simulink model "Control_ETHERLAB_2018b"  (R2018b)
settings: Solver=FixedStepDiscrete  StartTime=0.0  StopTime=inf  FixedStep=0.001  RelTol=1e-3
PreLoadFcn:
  | addpath(genpath('/opt/etherlab'))
InitFcn:
  | addpath(genpath('/opt/etherlab'))
undefined symbols (not defined in the file): motor_ec1
libraries: dspindex x10, dspfdesign x3
settings Model: SimulationMode=external  ExtModeTrigDuration=100  ExtModeArchiveFileName=measurement_data  ExtModeArchiveDirName=/home/cybathalon/Documents/Motor_test/Data/  Creator=schappler  LastModifiedBy=Rossgoderer
settings DataIOCC: SaveFormat=StructureWithTime  SaveOutput=off  SignalLogging=off  SaveTime=off
settings OptimizationCC: BlockReduction=off  ConditionallyExecuteInputs=off  OptimizeBlockIOStorage=off  BufferReuse=off  GlobalBufferReuse=off  ExpressionFolding=off  LocalBlockOutputs=off  OptimizeDataStoreBuffers=off  BusAssignmentInplaceUpdate=off
settings DebuggingCC: InheritedTsInSrcMsg=none
settings HardwareCC: ProdBitPerPointer=32  ProdBitPerSizeT=32  ProdBitPerPtrDiffT=32  ProdLargestAtomicInteger=Long  ProdWordSize=32  ProdHWDeviceType=ARM Compatible->ARM 10
settings SFSimCC: SimUseLocalCustomCode=off
settings RTWCC: Description=EtherLab PREEMT_RT Real-Time Target  SystemTargetFile=etherlab.tlc  PackageName=test  TemplateMakefile=etherlab_hrt.tmf  RTWUseLocalCustomCode=off
settings CodeAppCC: StateflowObjectComments=on
settings STFCustomTargetCC: TargetLangStandard=C99 (ISO)  GRTInterface=on  SystemTargetFile=etherlab.tlc
settings GRTTargetCC: ParMdlRefBuildCompliant=off  CompOptLevelCompliant=off  ConcurrentExecutionCompliant=off  CombineOutputUpdateFcns=off  MatFileLogging=off  CPPClassGenCompliant=off  GRTInterface=on  UseToolchainInfoCompliant=off  ExtMode=on  ExtModeStaticAlloc=on  ExtModeStaticAllocSize=10000000  ExtModeMexArgs='localhost' 0 17725  RTWCAPISignals=on  RTWCAPIParams=on
settings SimscapeCC: SimscapeNormalizeSystem=off

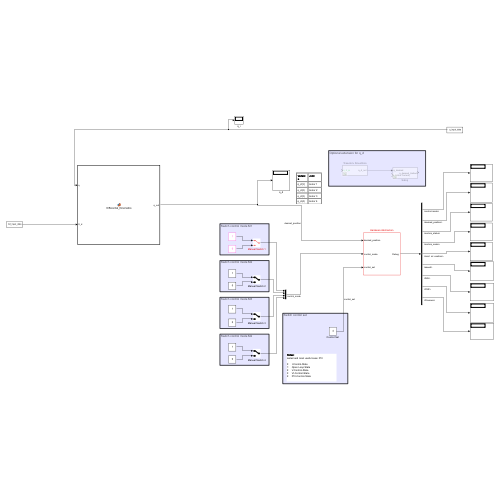
[thumbnail: Simulink's stored preview of the top-level diagram]
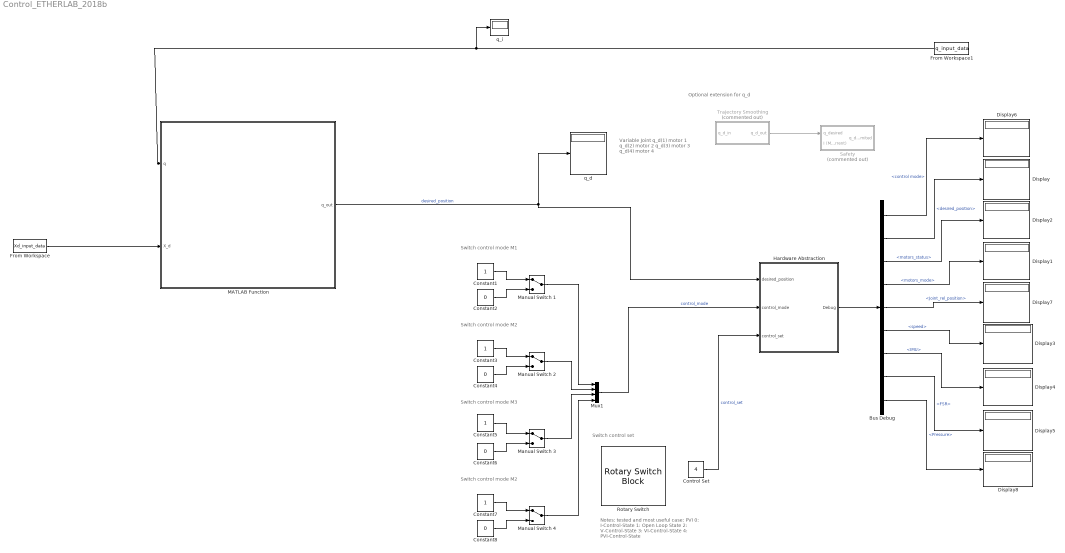
== system Control_ETHERLAB_2018b ==
  note: Optional extension for q_d
  note: Switch control mode M1
  note: Variable
      | Joint
      |
      | q_d(1)
      |
      | motor 1
      |
      | q_d(2)
      | motor 2
      |
      | q_d(3)
      | motor 3
      |
      | q_d(4)
      | motor 4
  note: Switch control mode M2
  note: Switch control mode M3
  note: Switch control mode M2
  note: Switch control set
  note: Notes:
      | tested and most useful case: PVI
      |
      | 0: I-Control-State
      | 1: Open Loop State
      | 2: V-Control-State
      | 3: VI-Control-State
      | 4: PVI-Control-State
  Bus Debug : BusSelector  OutputSignals=control mode,desired_position,motors_status,motors_mode,Joint_rel_position,speed,IMU,FSR,Pressure
  Constant{1,3,5,7} (4 alike) : Constant  VectorParams1D=off
  Constant{2,4,6,8} (4 alike) : Constant  Value=0  VectorParams1D=off
  Control Set : Constant  Value=4  VectorParams1D=off
  Display{,1..8} (9 alike) : Display
  From Workspace : FromWorkspace  VariableName=Xd_input_data  SampleTime=0.01  Interpolate=off  OutputAfterFinalValue=Setting to zero
  From Workspace1 : FromWorkspace  VariableName=q_input_data  SampleTime=0.01  Interpolate=off  OutputAfterFinalValue=Setting to zero
  Hardware Abstraction : Subsystem
  MATLAB Function : MATLAB Function  TreatAsAtomicUnit=on
  Manual Switch {1..4} (4 alike) : ManualSwitch
  Mux1 : Mux
  Rotary Switch : RotarySwitchBlock  WebBlockId=10885
      settings: Values={{'I', 'OL', 'V', 'VI', 'PVI'}, [0 1 2 3 4]}
  Safety : Subsystem  Commented=on
  Trajectory Smoothing : Subsystem  Commented=on
  q_d : Display
      settings: Description=|
      | Wrist
      | Gripper
  "q_i " : Display
      settings: Description=|
      | Wrist
      | Gripper
  wires:
  Trajectory Smoothing/1(q_d_out) -> Safety/1(q_desired)
  Hardware Abstraction/1("Debug ") -> Bus Debug/1
  Bus Debug/2 -> Display/1  "<desired_position>"
  Bus Debug/4 -> Display1/1  "<motors_mode>"
  Bus Debug/6 -> Display3/1  "<speed>"
  Bus Debug/1 -> Display6/1  "<control mode>"
  Bus Debug/5 -> Display7/1  "<Joint_rel_position>"
  Constant1/1 -> Manual Switch 1/1
  Constant2/1 -> Manual Switch 1/2
  Manual Switch 1/1 -> Mux1/1
  Mux1/1 -> Hardware Abstraction/2(control_mode)  "control_mode"
  Manual Switch 2/1 -> Mux1/2
  Constant4/1 -> Manual Switch 2/2
  Constant3/1 -> Manual Switch 2/1
  Constant5/1 -> Manual Switch 3/1
  Constant6/1 -> Manual Switch 3/2
  Manual Switch 3/1 -> Mux1/3
  Constant7/1 -> Manual Switch 4/1
  Constant8/1 -> Manual Switch 4/2
  Manual Switch 4/1 -> Mux1/4
  Control Set/1 -> Hardware Abstraction/3(control_set)  "control_set"
  Bus Debug/3 -> Display2/1  "<motors_status>"
  Bus Debug/7 -> Display4/1  "<IMU>"
  Bus Debug/8 -> Display5/1  "<FSR>"
  Bus Debug/9 -> Display8/1  "<Pressure>"
  MATLAB Function/1(q_out) -> Hardware Abstraction/1(desired_position), q_d/1  "desired_position"
  From Workspace/1 -> MATLAB Function/2(X_d)
  From Workspace1/1 -> "q_i "/1, MATLAB Function/1(q)

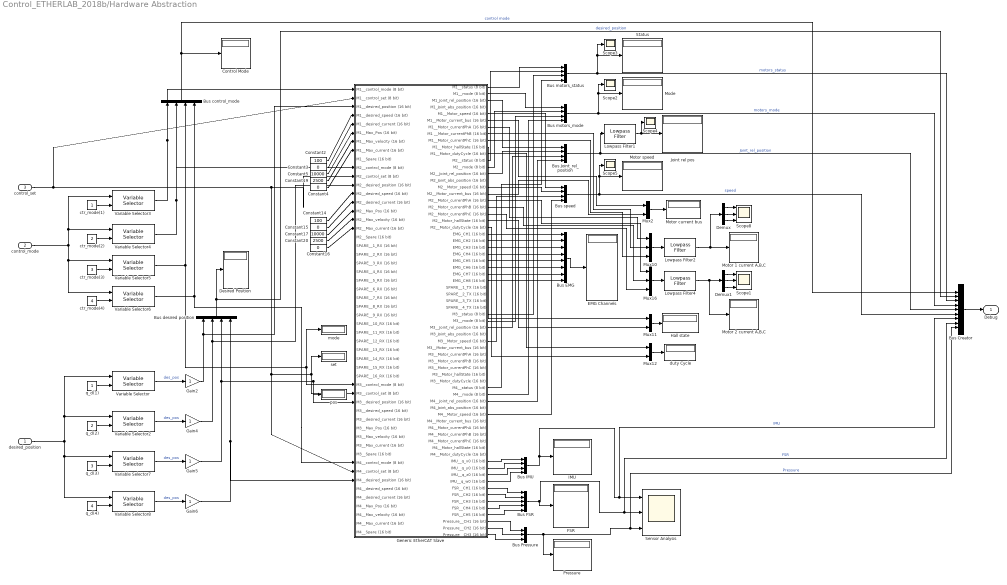
== system Control_ETHERLAB_2018b/Hardware Abstraction ==
  desired_position : Inport
  control_mode : Inport  Port=2
  control_set : Inport  Port=3
  Bus Creator : BusCreator  Inputs=9
  Bus EMG : BusCreator  Inputs=8
  Bus FSR : BusCreator  Inputs=5
  Bus IMU : BusCreator  Inputs=4
  Bus Joint_rel_position : BusCreator  Inputs=4
  Bus Pressure : BusCreator  Inputs=3
  Bus control_mode : BusCreator  Inputs=4
  Bus desired position : BusCreator  Inputs=4
  Bus motors_mode : BusCreator  Inputs=4
  Bus motors_status : BusCreator  Inputs=4
  Bus speed : BusCreator  Inputs=4
  Constant14 : Constant  Value=100
  Constant{3..4,15..16} (4 alike) : Constant  Value=0
  Constant17 : Constant  Value=10000
  Constant19 : Constant  Value=2500
  Constant2 : Constant  Value=100
  Constant20 : Constant  Value=2500
  Constant5 : Constant  Value=10000
  Control Mode : Display
  Demux : Demux  Outputs=3
  Demux1 : Demux  Outputs=3
  Desired Position : Display
  EMG Channels : Display
  FSR : Display
  Gain{2,4..6} (4 alike) : Gain
  Generic EtherCAT Slave : Subsystem
  Hall state : Display
  IMU : Display
  Joint rel pos : Display
  Lowpass Filter1 : dspfdesign/Lowpass Filter  FilterType=FIR  DesignForMinimumOrder=on  FilterOrder=50  PassbandFrequency=1  StopbandFrequency=10  PassbandRipple=0.1  StopbandAttenuation=10  InheritSampleRate=off  SampleRate=1000  SimulateUsing=Interpreted execution  roundingMode=Floor  coeffsDataTypeStr=fixdt(1,16)
  Lowpass Filter2 : dspfdesign/Lowpass Filter  FilterType=FIR  DesignForMinimumOrder=on  FilterOrder=50  PassbandFrequency=1  StopbandFrequency=10  PassbandRipple=0.1  StopbandAttenuation=80  InheritSampleRate=off  SampleRate=1000  SimulateUsing=Interpreted execution  roundingMode=Floor  coeffsDataTypeStr=fixdt(1,16)
  Lowpass Filter4 : dspfdesign/Lowpass Filter  FilterType=FIR  DesignForMinimumOrder=on  FilterOrder=50  PassbandFrequency=1  StopbandFrequency=10  PassbandRipple=0.1  StopbandAttenuation=80  InheritSampleRate=off  SampleRate=1000  SimulateUsing=Interpreted execution  roundingMode=Floor  coeffsDataTypeStr=fixdt(1,16)
  Mode : Display
  Motor 1 current A,B,C : Display
  Motor 2 current A,B,C : Display
  Motor current bus : Display
  Motor speed : Display
  Mux10 : Mux  Inputs=3
  Mux11 : Mux  Inputs=2
  Mux12 : Mux  Inputs=2
  Mux16 : Mux  Inputs=3
  Mux2 : Mux  Inputs=2
  Pressure : Display
  Scope1 : Scope  NumInputPorts=3
  Scope{2..5} (4 alike) : Scope
  Scope8 : Scope  NumInputPorts=3
  Sensor Analysis : Scope  NumInputPorts=3
  Status : Display
  Variable Selector{,2..8} (8 alike) : dspindex/Variable Selector  NumInputs=1  rowsOrCols=Rows  IdxMode=Variable  Elements=[1 3]  ZerOneIdxMode=One-based  errmode=Clip Index  FillMode=on  FillValues=0
  ctr_mode(1) : Constant  SampleTime=-1
  ctr_mode(2) : Constant  Value=2  SampleTime=-1
  ctr_mode(3) : Constant  Value=3  SampleTime=-1
  ctr_mode(4) : Constant  Value=4  SampleTime=-1
  duty Cycle : Display
  mode : Display
  pos : Display
  q_d(1) : Constant  SampleTime=-1
  q_d(2) : Constant  Value=2  SampleTime=-1
  q_d(3) : Constant  Value=3  SampleTime=-1
  q_d(4) : Constant  Value=4  SampleTime=-1
  "set " : Display
  "Debug " : Outport  VectorParamsAs1DForOutWhenUnconnected=off
  wires:
  Variable Selector/1 -> Gain2/1  "des_pos"
  q_d(1)/1 -> Variable Selector/2
  Bus motors_status/1 -> Scope3/1, Status/1, Bus Creator/3  "motors_status"
  Bus Creator/1 -> "Debug "/1
  q_d(2)/1 -> Variable Selector2/2
  Variable Selector2/1 -> Gain4/1  "des_pos"
  ctr_mode(1)/1 -> Variable Selector3/2
  ctr_mode(2)/1 -> Variable Selector4/2
  Bus EMG/1 -> EMG Channels/1
  Generic EtherCAT Slave/23(EMG_CH1 (16 bit)) -> Bus EMG/1
  Generic EtherCAT Slave/24(EMG_CH2 (16 bit)) -> Bus EMG/2
  Generic EtherCAT Slave/25(EMG_CH3 (16 bit)) -> Bus EMG/3
  Generic EtherCAT Slave/26(EMG_CH4 (16 bit)) -> Bus EMG/4
  Generic EtherCAT Slave/27(EMG_CH5 (16 bit)) -> Bus EMG/5
  Generic EtherCAT Slave/28(EMG_CH6 (16 bit)) -> Bus EMG/6
  Generic EtherCAT Slave/29(EMG_CH7 (16 bit)) -> Bus EMG/7
  Generic EtherCAT Slave/30(EMG_CH8 (16 bit)) -> Bus EMG/8
  Generic EtherCAT Slave/2(M1__mode (8 bit)) -> Bus motors_mode/1
  Generic EtherCAT Slave/1(M1__status (8 bit)) -> Bus motors_status/1
  Generic EtherCAT Slave/12(M2__status (8 bit)) -> Bus motors_status/2
  Generic EtherCAT Slave/13(M2__mode (8 bit)) -> Bus motors_mode/2
  Generic EtherCAT Slave/14(M2__Joint_rel_position (16 bit)) -> Bus Joint_rel_position/2
  Mux2/1 -> Motor current bus/1
  Mux10/1 -> Lowpass Filter2/1
  Generic EtherCAT Slave/6(M1__Motor_current_bus (16 bit)) -> Mux2/1
  Generic EtherCAT Slave/17(M2__Motor_current_bus (16 bit)) -> Mux2/2
  Generic EtherCAT Slave/7(M1__Motor_currentPhA (16 bit)) -> Mux10/1
  Generic EtherCAT Slave/8(M1 __Motor_currentPhB (16 bit)) -> Mux10/2
  Generic EtherCAT Slave/9(M1__Motor_currentPhC (16 bit)) -> Mux10/3
  Generic EtherCAT Slave/18(M2__Motor_currentPhA (16 bit)) -> Mux16/1
  Generic EtherCAT Slave/19(M2__Motor_currentPhB (16 bit)) -> Mux16/2
  Generic EtherCAT Slave/20(M2__Motor_currentPhC (16 bit)) -> Mux16/3
  Mux11/1 -> Hall state/1
  Generic EtherCAT Slave/10(M1__Motor_hallState (16 bit)) -> Mux11/1
  Generic EtherCAT Slave/21(M2__Motor_hallState (16 bit)) -> Mux11/2
  Mux12/1 -> duty Cycle/1
  Generic EtherCAT Slave/11(M1__Motor_dutyCycle (16 bit)) -> Mux12/1
  Generic EtherCAT Slave/22(M2__Motor_dutyCycle (16 bit)) -> Mux12/2
  Bus IMU/1 -> Sensor Analysis/1, Bus Creator/7, IMU/1  "IMU"
  Generic EtherCAT Slave/57(IMU__q_x0 (16 bit)) -> Bus IMU/1
  Generic EtherCAT Slave/58(IMU__q_y0 (16 bit)) -> Bus IMU/2
  Generic EtherCAT Slave/59(IMU__q_z0 (16 bit)) -> Bus IMU/3
  Generic EtherCAT Slave/60(IMU__q_w0 (16 bit)) -> Bus IMU/4
  Generic EtherCAT Slave/64(FSR__CH4 (16 bit)) -> Bus FSR/4
  Generic EtherCAT Slave/61(FSR__CH1 (16 bit)) -> Bus FSR/1
  Generic EtherCAT Slave/63(FSR__CH3 (16 bit)) -> Bus FSR/3
  Generic EtherCAT Slave/62(FSR__CH2 (16 bit)) -> Bus FSR/2
  Generic EtherCAT Slave/65(FSR__CH5 (16 bit)) -> Bus FSR/5
  Bus Pressure/1 -> Bus Creator/9, Sensor Analysis/3, Pressure/1  "Pressure"
  Generic EtherCAT Slave/66(Pressure__CH1 (16 bit)) -> Bus Pressure/1
  Generic EtherCAT Slave/67(Pressure__CH2 (16 bit)) -> Bus Pressure/2
  Generic EtherCAT Slave/68(Pressure__CH3 (16 bit)) -> Bus Pressure/3
  Variable Selector3/1 -> Generic EtherCAT Slave/1(M1__control_mode (8 bit)), Bus control_mode/1
  Constant14/1 -> Generic EtherCAT Slave/13(M2__desired_speed (16 bit))
  Constant15/1 -> Generic EtherCAT Slave/14(M2__desired_current (16 bit))
  Gain4/1 -> Generic EtherCAT Slave/12(M2__desired_position (16 bit)), Bus desired position/2
  Variable Selector4/1 -> Generic EtherCAT Slave/10(M2__control_mode (8 bit)), Bus control_mode/2
  control_set/1 -> Generic EtherCAT Slave/45(M4__control_set (8 bit)), "set "/1, Generic EtherCAT Slave/36(M3__control_set (8 bit)), Generic EtherCAT Slave/11(M2__control_set (8 bit)), Generic EtherCAT Slave/2(M1__control_set (8 bit))
  Constant2/1 -> Generic EtherCAT Slave/4(M1__desired_speed (16 bit))
  Constant19/1 -> Generic EtherCAT Slave/7(M1__Max_velocity (16 bit))
  Gain2/1 -> Generic EtherCAT Slave/3(M1__desired_position (16 bit)), Bus desired position/1
  Constant5/1 -> Generic EtherCAT Slave/6(M1__Max_Pos (16 bit))
  Constant3/1 -> Generic EtherCAT Slave/5(M1__desired_current (16 bit))
  Constant4/1 -> Generic EtherCAT Slave/8(M1__Max_current (16 bit))
  Lowpass Filter2/1 -> Demux/1, Motor 1 current A,B,C/1
  Mux16/1 -> Lowpass Filter4/1
  Lowpass Filter4/1 -> Demux1/1, Motor 2 current A,B,C/1
  ctr_mode(3)/1 -> Variable Selector5/2
  ctr_mode(4)/1 -> Variable Selector6/2
  control_mode/1 -> Variable Selector3/1, Variable Selector4/1, Variable Selector6/1, Variable Selector5/1
  Variable Selector5/1 -> Bus control_mode/3, mode/1, Generic EtherCAT Slave/35(M3__control_mode (8 bit))
  Variable Selector6/1 -> Bus control_mode/4, Generic EtherCAT Slave/44(M4__control_mode (8 bit))
  Bus control_mode/1 -> Bus Creator/1, Control Mode/1  "control mode"
  q_d(3)/1 -> Variable Selector7/2
  desired_position/1 -> Variable Selector2/1, Variable Selector/1, Variable Selector8/1, Variable Selector7/1
  q_d(4)/1 -> Variable Selector8/2
  Variable Selector7/1 -> Gain5/1  "des_pos"
  Variable Selector8/1 -> Gain6/1  "des_pos"
  Gain5/1 -> pos/1, Generic EtherCAT Slave/37(M3__desired_position (16 bit)), Bus desired position/3
  Gain6/1 -> Generic EtherCAT Slave/46(M4__desired_position (16 bit)), Bus desired position/4
  Bus desired position/1 -> Desired Position/1, Bus Creator/2  "desired_position"
  Demux/1 -> Scope8/1
  Demux/2 -> Scope8/2
  Demux/3 -> Scope8/3
  Demux1/3 -> Scope1/3
  Demux1/2 -> Scope1/2
  Demux1/1 -> Scope1/1
  Generic EtherCAT Slave/35(M3__status (8 bit)) -> Bus motors_status/3
  Generic EtherCAT Slave/46(M4__status (8 bit)) -> Bus motors_status/4
  Generic EtherCAT Slave/36(M3__mode (8 bit)) -> Bus motors_mode/3
  Generic EtherCAT Slave/47(M4__mode (8 bit)) -> Bus motors_mode/4
  Bus motors_mode/1 -> Bus Creator/4, Scope2/1, Mode/1  "motors_mode"
  Generic EtherCAT Slave/3(M1_Joint_rel_position (16 bit)) -> Bus Joint_rel_position/1
  Generic EtherCAT Slave/37(M3__Joint_rel_position (16 bit)) -> Bus Joint_rel_position/3
  Generic EtherCAT Slave/48(M4__Joint_rel_position (16 bit)) -> Bus Joint_rel_position/4
  Bus Joint_rel_position/1 -> Lowpass Filter1/1, Bus Creator/5  "Joint_rel_position"
  Bus speed/1 -> Bus Creator/6, Scope5/1, Motor speed/1  "speed"
  Generic EtherCAT Slave/5(M1__Motor_speed (16 bit)) -> Bus speed/1
  Generic EtherCAT Slave/16(M2__Motor_speed (16 bit)) -> Bus speed/2
  Generic EtherCAT Slave/39(M3__Motor_speed (16 bit)) -> Bus speed/3
  Generic EtherCAT Slave/50(M4__Motor_speed (16 bit)) -> Bus speed/4
  Bus FSR/1 -> Sensor Analysis/2, Bus Creator/8, FSR/1  "FSR"
  Constant17/1 -> Generic EtherCAT Slave/15(M2__Max_Pos (16 bit))
  Constant20/1 -> Generic EtherCAT Slave/16(M2__Max_velocity (16 bit))
  Constant16/1 -> Generic EtherCAT Slave/17(M2__Max_current (16 bit))
  Lowpass Filter1/1 -> Scope4/1, Joint rel pos/1

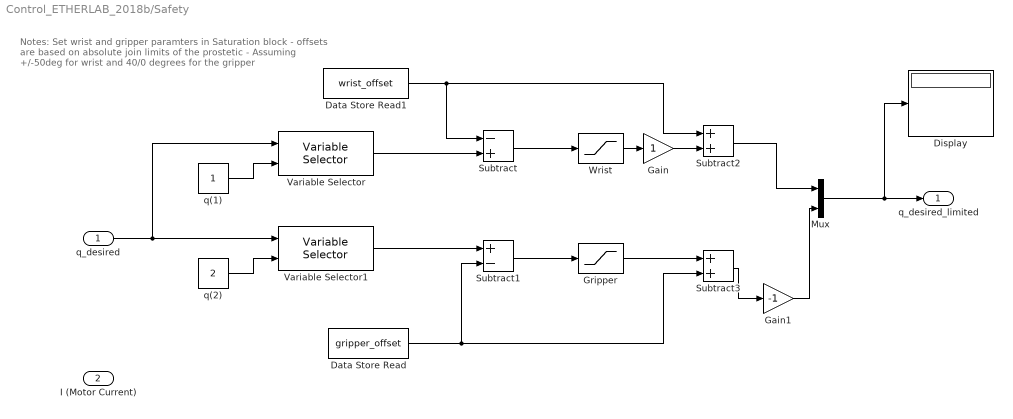
== system Control_ETHERLAB_2018b/Safety ==
  note: Notes:
      | Set wrist and gripper paramters in Saturation block
      | - offsets are based on absolute join limits of the prostetic
      | - Assuming +/-50deg for wrist and 40/0 degrees for the gripper
  q_desired : Inport
  I (Motor Current) : Inport  Port=2
  Data Store Read : DataStoreRead  DataStoreName=gripper_offset  DataStoreElements=gripper_offset
  Data Store Read1 : DataStoreRead  DataStoreName=wrist_offset  DataStoreElements=wrist_offset
  Display : Display
  Gain : Gain
  Gain1 : Gain  Gain=-1
  Gripper : Saturate  UpperLimit=40  LowerLimit=-10
  Mux : Mux  Inputs=2
  Subtract : Sum  Inputs=-+
  Subtract1 : Sum  Inputs=+-
  Subtract2 : Sum
  Subtract3 : Sum
  Variable Selector : dspindex/Variable Selector  NumInputs=1  rowsOrCols=Rows  IdxMode=Variable  Elements=[1 3]  ZerOneIdxMode=One-based  errmode=Clip Index  FillMode=on  FillValues=0
  Variable Selector1 : dspindex/Variable Selector  NumInputs=1  rowsOrCols=Rows  IdxMode=Variable  Elements=[1 3]  ZerOneIdxMode=One-based  errmode=Clip Index  FillMode=on  FillValues=0
  Wrist : Saturate  UpperLimit=100  LowerLimit=-100
  q(1) : Constant  SampleTime=-1
  q(2) : Constant  Value=2  SampleTime=-1
  q_desired_limited : Outport  VectorParamsAs1DForOutWhenUnconnected=off
  wires:
  q(1)/1 -> Variable Selector/2
  q_desired/1 -> Variable Selector1/1, Variable Selector/1
  q(2)/1 -> Variable Selector1/2
  Mux/1 -> Display/1, q_desired_limited/1
  Variable Selector/1 -> Subtract/2
  Subtract/1 -> Wrist/1
  Subtract1/1 -> Gripper/1
  Variable Selector1/1 -> Subtract1/1
  Data Store Read/1 -> Subtract3/2, Subtract1/2
  Data Store Read1/1 -> Subtract2/1, Subtract/1
  Wrist/1 -> Gain/1
  Subtract2/1 -> Mux/1
  Subtract3/1 -> Gain1/1
  Gain/1 -> Subtract2/2
  Gripper/1 -> Subtract3/1
  Gain1/1 -> Mux/2

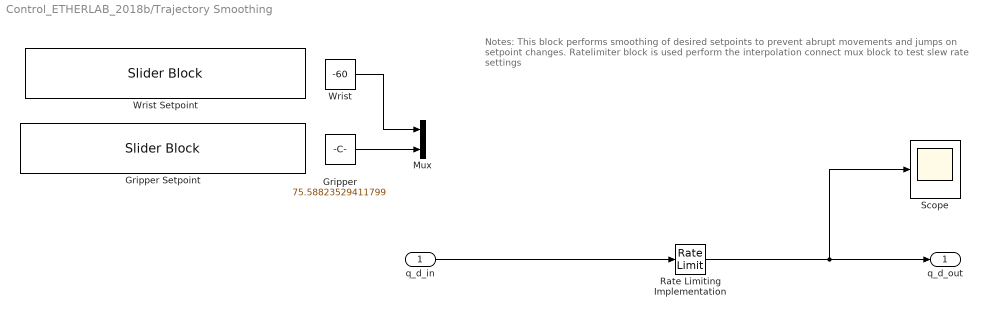
== system Control_ETHERLAB_2018b/Trajectory Smoothing ==
  note: Notes:
      | This block performs smoothing of desired setpoints to prevent abrupt movements and jumps on setpoint changes.
      | Ratelimiter block is used perform the interpolation
      |
      | connect mux block to test slew rate settings
  q_d_in : Inport
  Gripper : Constant  Value=75.58823529411799
  Gripper Setpoint : SliderBlock  ScaleMin=-120  ScaleMax=120
  Mux : Mux  Inputs=2
  Rate Limiting Implementation : RateLimiter  RisingSlewLimit=40  FallingSlewLimit=-40  SampleTimeMode=inherited
  Scope : Scope
  Wrist : Constant  Value=-60
  Wrist Setpoint : SliderBlock  ScaleMin=-120  ScaleMax=120
  q_d_out : Outport  VectorParamsAs1DForOutWhenUnconnected=off
  wires:
  Gripper/1 -> Mux/2
  Wrist/1 -> Mux/1
  q_d_in/1 -> Rate Limiting Implementation/1
  Rate Limiting Implementation/1 -> Scope/1, q_d_out/1

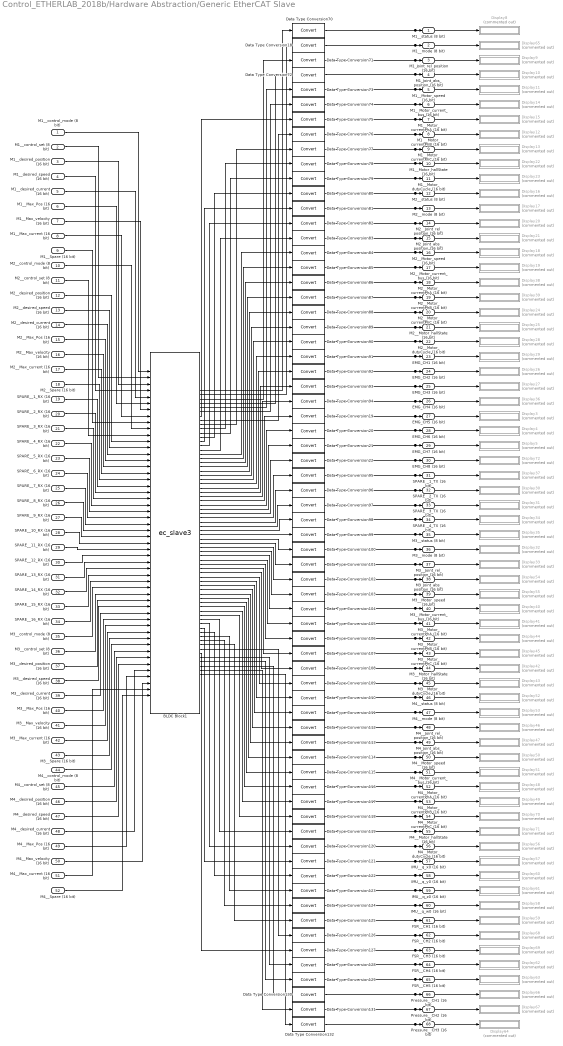
== system Control_ETHERLAB_2018b/Hardware Abstraction/Generic EtherCAT Slave ==
  M1__control_mode (8 bit) : Inport
  M1__control_set (8 bit) : Inport  Port=2
  M1__desired_position (16 bit) : Inport  Port=3
  M1__desired_speed (16 bit) : Inport  Port=4
  M1__desired_current (16 bit) : Inport  Port=5
  M1__Max_Pos (16 bit) : Inport  Port=6
  M1__Max_velocity (16 bit) : Inport  Port=7
  M1__Max_current (16 bit) : Inport  Port=8
  M1__Spare (16 bit) : Inport  Port=9
  M2__control_mode (8 bit) : Inport  Port=10
  M2__control_set (8 bit) : Inport  Port=11
  M2__desired_position (16 bit) : Inport  Port=12
  M2__desired_speed (16 bit) : Inport  Port=13
  M2__desired_current (16 bit) : Inport  Port=14
  M2__Max_Pos (16 bit) : Inport  Port=15
  M2__Max_velocity (16 bit) : Inport  Port=16
  M2__Max_current (16 bit) : Inport  Port=17
  M2__Spare (16 bit) : Inport  Port=18
  SPARE__1_RX (16 bit) : Inport  Port=19
  SPARE__2_RX (16 bit) : Inport  Port=20
  SPARE__3_RX (16 bit) : Inport  Port=21
  SPARE__4_RX (16 bit) : Inport  Port=22
  SPARE__5_RX (16 bit) : Inport  Port=23
  SPARE__6_RX (16 bit) : Inport  Port=24
  SPARE__7_RX (16 bit) : Inport  Port=25
  SPARE__8_RX (16 bit) : Inport  Port=26
  SPARE__9_RX (16 bit) : Inport  Port=27
  SPARE__10_RX (16 bit) : Inport  Port=28
  SPARE__11_RX (16 bit) : Inport  Port=29
  SPARE__12_RX (16 bit) : Inport  Port=30
  SPARE__13_RX (16 bit) : Inport  Port=31
  SPARE__14_RX (16 bit) : Inport  Port=32
  SPARE__15_RX (16 bit) : Inport  Port=33
  SPARE__16_RX (16 bit) : Inport  Port=34
  M3__control_mode (8 bit) : Inport  Port=35
  M3__control_set (8 bit) : Inport  Port=36
  M3__desired_position (16 bit) : Inport  Port=37
  M3__desired_speed (16 bit) : Inport  Port=38
  M3__desired_current (16 bit) : Inport  Port=39
  M3__Max_Pos (16 bit) : Inport  Port=40
  M3__Max_velocity (16 bit) : Inport  Port=41
  M3__Max_current (16 bit) : Inport  Port=42
  M3__Spare (16 bit) : Inport  Port=43
  M4__control_mode (8 bit) : Inport  Port=44
  M4__control_set (8 bit) : Inport  Port=45
  M4__desired_position (16 bit) : Inport  Port=46
  M4__desired_speed (16 bit) : Inport  Port=47
  M4__desired_current (16 bit) : Inport  Port=48
  M4__Max_Pos (16 bit) : Inport  Port=49
  M4__Max_velocity (16 bit) : Inport  Port=50
  M4__Max_current (16 bit) : Inport  Port=51
  M4__Spare (16 bit) : Inport  Port=52
  BLDC Block1 : S-Function  AncestorBlock=etherlab_lib/EtherCAT/Generic_0  FunctionName=ec_slave3  Parameters=Address,rv.SlaveConfig,rv.PortConfig,debug,tsample  SFunctionModules='ecrt_support'  SFunctionDeploymentMode=off  EnableBusSupport=off  mask(Generic EtherCAT Slave){master=0, index=0, rv=motor_ec1, tsample=-1, debug=0}
      mask prompts: index "Slave Index"; rv "EtherCAT Slave Configuration struct. (SlaveConfig, PortConfig)"; tsample "Sample Time"
      mask help:
      | The generic EtherCAT Slave is used to create any slave not contained
      | in this library. A mask input variable, <b>EtherCAT Slave Configuration</b>,
      | has to be set up by the user. This configures the slave.
      mask init:
      | Address = EtherCATSlave.formatAddress(master,index,tsample);
      | 
      | if ~isfield(rv,'PortConfig') || isempty(rv)
      |    rv.PortConfig = [];
      | end
      | 
      | if ~isfield(rv,'SlaveConfig') || isempty(rv)
      |    rv.SlaveConfig = [];
      | end
      | 
      | if ~isfield(rv.SlaveConfig,'description') || isempty(rv)
      |    slave_name = 'unknown';
      | else
      |    slave_name = rv.SlaveConfig.description;
      | end
      mask Help: web(etherlab_help_path('generic.html'), '-helpbrowser');
      mask Display:
      | fprintf('Generic Slave\n%s \n%i Idx:%s', ...
      |     slave_name, master, mat2str(index))
  Data Type Conversion{18..22,70..132} (68 alike) : DataTypeConversion
  Display{3..5,8..72} (68 alike) : Display  Commented=on
  M1__status (8 bit) : Outport  VectorParamsAs1DForOutWhenUnconnected=off
  M1__mode (8 bit) : Outport  Port=2  VectorParamsAs1DForOutWhenUnconnected=off
  M1_Joint_rel_position (16 bit) : Outport  Port=3  VectorParamsAs1DForOutWhenUnconnected=off
  M1_Joint_abs_position (16 bit) : Outport  Port=4  VectorParamsAs1DForOutWhenUnconnected=off
  M1__Motor_speed (16 bit) : Outport  Port=5  VectorParamsAs1DForOutWhenUnconnected=off
  M1__Motor_current_bus (16 bit) : Outport  Port=6  VectorParamsAs1DForOutWhenUnconnected=off
  M1__Motor_currentPhA (16 bit) : Outport  Port=7  VectorParamsAs1DForOutWhenUnconnected=off
  M1 __Motor_currentPhB (16 bit) : Outport  Port=8  VectorParamsAs1DForOutWhenUnconnected=off
  M1__Motor_currentPhC (16 bit) : Outport  Port=9  VectorParamsAs1DForOutWhenUnconnected=off
  M1__Motor_hallState (16 bit) : Outport  Port=10  VectorParamsAs1DForOutWhenUnconnected=off
  M1__Motor_dutyCycle (16 bit) : Outport  Port=11  VectorParamsAs1DForOutWhenUnconnected=off
  M2__status (8 bit) : Outport  Port=12  VectorParamsAs1DForOutWhenUnconnected=off
  M2__mode (8 bit) : Outport  Port=13  VectorParamsAs1DForOutWhenUnconnected=off
  M2__Joint_rel_position (16 bit) : Outport  Port=14  VectorParamsAs1DForOutWhenUnconnected=off
  M2_Joint_abs_position (16 bit) : Outport  Port=15  VectorParamsAs1DForOutWhenUnconnected=off
  M2__Motor_speed (16 bit) : Outport  Port=16  VectorParamsAs1DForOutWhenUnconnected=off
  M2__Motor_current_bus (16 bit) : Outport  Port=17  VectorParamsAs1DForOutWhenUnconnected=off
  M2__Motor_currentPhA (16 bit) : Outport  Port=18  VectorParamsAs1DForOutWhenUnconnected=off
  M2__Motor_currentPhB (16 bit) : Outport  Port=19  VectorParamsAs1DForOutWhenUnconnected=off
  M2__Motor_currentPhC (16 bit) : Outport  Port=20  VectorParamsAs1DForOutWhenUnconnected=off
  M2__Motor_hallState (16 bit) : Outport  Port=21  VectorParamsAs1DForOutWhenUnconnected=off
  M2__Motor_dutyCycle (16 bit) : Outport  Port=22  VectorParamsAs1DForOutWhenUnconnected=off
  EMG_CH1 (16 bit) : Outport  Port=23  VectorParamsAs1DForOutWhenUnconnected=off
  EMG_CH2 (16 bit) : Outport  Port=24  VectorParamsAs1DForOutWhenUnconnected=off
  EMG_CH3 (16 bit) : Outport  Port=25  VectorParamsAs1DForOutWhenUnconnected=off
  EMG_CH4 (16 bit) : Outport  Port=26  VectorParamsAs1DForOutWhenUnconnected=off
  EMG_CH5 (16 bit) : Outport  Port=27  VectorParamsAs1DForOutWhenUnconnected=off
  EMG_CH6 (16 bit) : Outport  Port=28  VectorParamsAs1DForOutWhenUnconnected=off
  EMG_CH7 (16 bit) : Outport  Port=29  VectorParamsAs1DForOutWhenUnconnected=off
  EMG_CH8 (16 bit) : Outport  Port=30  VectorParamsAs1DForOutWhenUnconnected=off
  SPARE__1_TX (16 bit) : Outport  Port=31  VectorParamsAs1DForOutWhenUnconnected=off
  SPARE__2_TX (16 bit) : Outport  Port=32  VectorParamsAs1DForOutWhenUnconnected=off
  SPARE__3_TX (16 bit) : Outport  Port=33  VectorParamsAs1DForOutWhenUnconnected=off
  SPARE__4_TX (16 bit) : Outport  Port=34  VectorParamsAs1DForOutWhenUnconnected=off
  M3__status (8 bit) : Outport  Port=35  VectorParamsAs1DForOutWhenUnconnected=off
  M3__mode (8 bit) : Outport  Port=36  VectorParamsAs1DForOutWhenUnconnected=off
  M3__Joint_rel_position (16 bit) : Outport  Port=37  VectorParamsAs1DForOutWhenUnconnected=off
  M3_Joint_abs_position (16 bit) : Outport  Port=38  VectorParamsAs1DForOutWhenUnconnected=off
  M3__Motor_speed (16 bit) : Outport  Port=39  VectorParamsAs1DForOutWhenUnconnected=off
  M3__Motor_current_bus (16 bit) : Outport  Port=40  VectorParamsAs1DForOutWhenUnconnected=off
  M3__Motor_currentPhA (16 bit) : Outport  Port=41  VectorParamsAs1DForOutWhenUnconnected=off
  M3__Motor_currentPhB (16 bit) : Outport  Port=42  VectorParamsAs1DForOutWhenUnconnected=off
  M3__Motor_currentPhC (16 bit) : Outport  Port=43  VectorParamsAs1DForOutWhenUnconnected=off
  M3__Motor_hallState (16 bit) : Outport  Port=44  VectorParamsAs1DForOutWhenUnconnected=off
  M3__Motor_dutyCycle (16 bit) : Outport  Port=45  VectorParamsAs1DForOutWhenUnconnected=off
  M4__status (8 bit) : Outport  Port=46  VectorParamsAs1DForOutWhenUnconnected=off
  M4__mode (8 bit) : Outport  Port=47  VectorParamsAs1DForOutWhenUnconnected=off
  M4__Joint_rel_position (16 bit) : Outport  Port=48  VectorParamsAs1DForOutWhenUnconnected=off
  M4_Joint_abs_position (16 bit) : Outport  Port=49  VectorParamsAs1DForOutWhenUnconnected=off
  M4__Motor_speed (16 bit) : Outport  Port=50  VectorParamsAs1DForOutWhenUnconnected=off
  M4__Motor_current_bus (16 bit) : Outport  Port=51  VectorParamsAs1DForOutWhenUnconnected=off
  M4__Motor_currentPhA (16 bit) : Outport  Port=52  VectorParamsAs1DForOutWhenUnconnected=off
  M4__Motor_currentPhB (16 bit) : Outport  Port=53  VectorParamsAs1DForOutWhenUnconnected=off
  M4__Motor_currentPhC (16 bit) : Outport  Port=54  VectorParamsAs1DForOutWhenUnconnected=off
  M4__Motor_hallState (16 bit) : Outport  Port=55  VectorParamsAs1DForOutWhenUnconnected=off
  M4__Motor_dutyCycle (16 bit) : Outport  Port=56  VectorParamsAs1DForOutWhenUnconnected=off
  IMU__q_x0 (16 bit) : Outport  Port=57  VectorParamsAs1DForOutWhenUnconnected=off
  IMU__q_y0 (16 bit) : Outport  Port=58  VectorParamsAs1DForOutWhenUnconnected=off
  IMU__q_z0 (16 bit) : Outport  Port=59  VectorParamsAs1DForOutWhenUnconnected=off
  IMU__q_w0 (16 bit) : Outport  Port=60  VectorParamsAs1DForOutWhenUnconnected=off
  FSR__CH1 (16 bit) : Outport  Port=61  VectorParamsAs1DForOutWhenUnconnected=off
  FSR__CH2 (16 bit) : Outport  Port=62  VectorParamsAs1DForOutWhenUnconnected=off
  FSR__CH3 (16 bit) : Outport  Port=63  VectorParamsAs1DForOutWhenUnconnected=off
  FSR__CH4 (16 bit) : Outport  Port=64  VectorParamsAs1DForOutWhenUnconnected=off
  FSR__CH5 (16 bit) : Outport  Port=65  VectorParamsAs1DForOutWhenUnconnected=off
  Pressure__CH1 (16 bit) : Outport  Port=66  VectorParamsAs1DForOutWhenUnconnected=off
  Pressure__CH2 (16 bit) : Outport  Port=67  VectorParamsAs1DForOutWhenUnconnected=off
  Pressure__CH3 (16 bit) : Outport  Port=68  VectorParamsAs1DForOutWhenUnconnected=off
  wires:
  M1__control_mode (8 bit)/1 -> BLDC Block1/1
  M1__control_set (8 bit)/1 -> BLDC Block1/2
  M1__desired_position (16 bit)/1 -> BLDC Block1/3
  M1__desired_speed (16 bit)/1 -> BLDC Block1/4
  M1__desired_current (16 bit)/1 -> BLDC Block1/5
  M1__Max_Pos (16 bit)/1 -> BLDC Block1/6
  M1__Max_velocity (16 bit)/1 -> BLDC Block1/7
  M1__Max_current (16 bit)/1 -> BLDC Block1/8
  M1__Spare (16 bit)/1 -> BLDC Block1/9
  M2__control_mode (8 bit)/1 -> BLDC Block1/10
  M2__control_set (8 bit)/1 -> BLDC Block1/11
  M2__desired_position (16 bit)/1 -> BLDC Block1/12
  M2__desired_speed (16 bit)/1 -> BLDC Block1/13
  M2__desired_current (16 bit)/1 -> BLDC Block1/14
  M2__Max_Pos (16 bit)/1 -> BLDC Block1/15
  M2__Max_velocity (16 bit)/1 -> BLDC Block1/16
  M2__Max_current (16 bit)/1 -> BLDC Block1/17
  M2__Spare (16 bit)/1 -> BLDC Block1/18
  SPARE__1_RX (16 bit)/1 -> BLDC Block1/19
  SPARE__2_RX (16 bit)/1 -> BLDC Block1/20
  SPARE__3_RX (16 bit)/1 -> BLDC Block1/21
  SPARE__4_RX (16 bit)/1 -> BLDC Block1/22
  SPARE__5_RX (16 bit)/1 -> BLDC Block1/23
  SPARE__6_RX (16 bit)/1 -> BLDC Block1/24
  SPARE__7_RX (16 bit)/1 -> BLDC Block1/25
  SPARE__8_RX (16 bit)/1 -> BLDC Block1/26
  SPARE__9_RX (16 bit)/1 -> BLDC Block1/27
  SPARE__10_RX (16 bit)/1 -> BLDC Block1/28
  SPARE__11_RX (16 bit)/1 -> BLDC Block1/29
  SPARE__12_RX (16 bit)/1 -> BLDC Block1/30
  SPARE__13_RX (16 bit)/1 -> BLDC Block1/31
  SPARE__14_RX (16 bit)/1 -> BLDC Block1/32
  SPARE__15_RX (16 bit)/1 -> BLDC Block1/33
  SPARE__16_RX (16 bit)/1 -> BLDC Block1/34
  M3__control_mode (8 bit)/1 -> BLDC Block1/35
  M3__control_set (8 bit)/1 -> BLDC Block1/36
  M3__desired_position (16 bit)/1 -> BLDC Block1/37
  M3__desired_speed (16 bit)/1 -> BLDC Block1/38
  M3__desired_current (16 bit)/1 -> BLDC Block1/39
  M3__Max_Pos (16 bit)/1 -> BLDC Block1/40
  M3__Max_velocity (16 bit)/1 -> BLDC Block1/41
  M3__Max_current (16 bit)/1 -> BLDC Block1/42
  M3__Spare (16 bit)/1 -> BLDC Block1/43
  M4__control_mode (8 bit)/1 -> BLDC Block1/44
  M4__control_set (8 bit)/1 -> BLDC Block1/45
  M4__desired_position (16 bit)/1 -> BLDC Block1/46
  M4__desired_speed (16 bit)/1 -> BLDC Block1/47
  M4__desired_current (16 bit)/1 -> BLDC Block1/48
  M4__Max_Pos (16 bit)/1 -> BLDC Block1/49
  M4__Max_velocity (16 bit)/1 -> BLDC Block1/50
  M4__Max_current (16 bit)/1 -> BLDC Block1/51
  M4__Spare (16 bit)/1 -> BLDC Block1/52
  BLDC Block1/1 -> Data Type Conversion70/1
  BLDC Block1/3 -> Data Type Conversion71/1
  BLDC Block1/4 -> Data Type Conversion72/1
  BLDC Block1/5 -> Data Type Conversion73/1
  BLDC Block1/6 -> Data Type Conversion74/1
  BLDC Block1/7 -> Data Type Conversion75/1
  BLDC Block1/8 -> Data Type Conversion76/1
  BLDC Block1/9 -> Data Type Conversion77/1
  BLDC Block1/10 -> Data Type Conversion78/1
  BLDC Block1/11 -> Data Type Conversion79/1
  BLDC Block1/12 -> Data Type Conversion80/1
  BLDC Block1/13 -> Data Type Conversion81/1
  BLDC Block1/14 -> Data Type Conversion82/1
  BLDC Block1/15 -> Data Type Conversion83/1
  BLDC Block1/16 -> Data Type Conversion84/1
  BLDC Block1/17 -> Data Type Conversion85/1
  BLDC Block1/18 -> Data Type Conversion86/1
  BLDC Block1/19 -> Data Type Conversion87/1
  BLDC Block1/20 -> Data Type Conversion88/1
  BLDC Block1/21 -> Data Type Conversion89/1
  BLDC Block1/22 -> Data Type Conversion90/1
  BLDC Block1/23 -> Data Type Conversion91/1
  BLDC Block1/24 -> Data Type Conversion92/1
  BLDC Block1/25 -> Data Type Conversion93/1
  BLDC Block1/26 -> Data Type Conversion94/1
  BLDC Block1/31 -> Data Type Conversion95/1
  BLDC Block1/32 -> Data Type Conversion96/1
  BLDC Block1/33 -> Data Type Conversion97/1
  BLDC Block1/34 -> Data Type Conversion98/1
  BLDC Block1/35 -> Data Type Conversion99/1
  BLDC Block1/36 -> Data Type Conversion100/1
  BLDC Block1/37 -> Data Type Conversion101/1
  BLDC Block1/38 -> Data Type Conversion102/1
  BLDC Block1/39 -> Data Type Conversion103/1
  BLDC Block1/40 -> Data Type Conversion104/1
  BLDC Block1/41 -> Data Type Conversion105/1
  BLDC Block1/42 -> Data Type Conversion106/1
  BLDC Block1/43 -> Data Type Conversion107/1
  BLDC Block1/44 -> Data Type Conversion108/1
  BLDC Block1/45 -> Data Type Conversion109/1
  BLDC Block1/46 -> Data Type Conversion110/1
  BLDC Block1/47 -> Data Type Conversion111/1
  BLDC Block1/48 -> Data Type Conversion112/1
  BLDC Block1/49 -> Data Type Conversion113/1
  BLDC Block1/50 -> Data Type Conversion114/1
  BLDC Block1/51 -> Data Type Conversion115/1
  BLDC Block1/52 -> Data Type Conversion116/1
  BLDC Block1/53 -> Data Type Conversion117/1
  BLDC Block1/54 -> Data Type Conversion118/1
  BLDC Block1/55 -> Data Type Conversion119/1
  BLDC Block1/56 -> Data Type Conversion120/1
  BLDC Block1/57 -> Data Type Conversion121/1
  BLDC Block1/58 -> Data Type Conversion122/1
  BLDC Block1/59 -> Data Type Conversion123/1
  BLDC Block1/60 -> Data Type Conversion124/1
  BLDC Block1/61 -> Data Type Conversion125/1
  BLDC Block1/62 -> Data Type Conversion126/1
  BLDC Block1/63 -> Data Type Conversion127/1
  BLDC Block1/64 -> Data Type Conversion128/1
  BLDC Block1/65 -> Data Type Conversion129/1
  BLDC Block1/66 -> Data Type Conversion130/1
  BLDC Block1/67 -> Data Type Conversion131/1
  BLDC Block1/68 -> Data Type Conversion132/1
  Data Type Conversion70/1 -> Display8/1, M1__status (8 bit)/1
  Data Type Conversion74/1 -> Display14/1, M1__Motor_current_bus (16 bit)/1
  Data Type Conversion77/1 -> Display13/1, M1__Motor_currentPhC (16 bit)/1
  Data Type Conversion75/1 -> Display15/1, M1__Motor_currentPhA (16 bit)/1
  Data Type Conversion78/1 -> Display22/1, M1__Motor_hallState (16 bit)/1
  Data Type Conversion76/1 -> Display12/1, M1 __Motor_currentPhB (16 bit)/1
  Data Type Conversion79/1 -> Display23/1, M1__Motor_dutyCycle (16 bit)/1
  Data Type Conversion85/1 -> Display19/1, M2__Motor_current_bus (16 bit)/1
  Data Type Conversion81/1 -> Display17/1, M2__mode (8 bit)/1
  Data Type Conversion84/1 -> Display18/1, M2__Motor_speed (16 bit)/1
  Data Type Conversion87/1 -> Display39/1, M2__Motor_currentPhB (16 bit)/1
  Data Type Conversion86/1 -> Display38/1, M2__Motor_currentPhA (16 bit)/1
  Data Type Conversion83/1 -> Display21/1, M2_Joint_abs_position (16 bit)/1
  Data Type Conversion89/1 -> Display25/1, M2__Motor_hallState (16 bit)/1
  Data Type Conversion82/1 -> Display20/1, M2__Joint_rel_position (16 bit)/1
  Data Type Conversion80/1 -> Display16/1, M2__status (8 bit)/1
  Data Type Conversion88/1 -> Display24/1, M2__Motor_currentPhC (16 bit)/1
  Data Type Conversion96/1 -> SPARE__2_TX (16 bit)/1, Display30/1
  Data Type Conversion93/1 -> Display27/1, EMG_CH3 (16 bit)/1
  Data Type Conversion92/1 -> Display26/1, EMG_CH2 (16 bit)/1
  Data Type Conversion95/1 -> SPARE__1_TX (16 bit)/1, Display37/1
  Data Type Conversion99/1 -> M3__status (8 bit)/1, Display35/1
  Data Type Conversion90/1 -> Display28/1, M2__Motor_dutyCycle (16 bit)/1
  Data Type Conversion91/1 -> Display29/1, EMG_CH1 (16 bit)/1
  Data Type Conversion94/1 -> Display36/1, EMG_CH4 (16 bit)/1
  Data Type Conversion98/1 -> SPARE__4_TX (16 bit)/1, Display34/1
  Data Type Conversion101/1 -> Display33/1, M3__Joint_rel_position (16 bit)/1
  Data Type Conversion105/1 -> M3__Motor_currentPhA (16 bit)/1, Display41/1
  Data Type Conversion103/1 -> M3__Motor_speed (16 bit)/1, Display55/1
  Data Type Conversion102/1 -> Display54/1, M3_Joint_abs_position (16 bit)/1
  Data Type Conversion104/1 -> M3__Motor_current_bus (16 bit)/1, Display40/1
  Data Type Conversion108/1 -> Display42/1, M3__Motor_hallState (16 bit)/1
  Data Type Conversion107/1 -> Display45/1, M3__Motor_currentPhC (16 bit)/1
  Data Type Conversion106/1 -> Display44/1, M3__Motor_currentPhB (16 bit)/1
  Data Type Conversion109/1 -> Display43/1, M3__Motor_dutyCycle (16 bit)/1
  Data Type Conversion112/1 -> M4__Joint_rel_position (16 bit)/1, Display46/1
  Data Type Conversion115/1 -> Display51/1, M4__Motor_current_bus (16 bit)/1
  Data Type Conversion117/1 -> Display49/1, M4__Motor_currentPhB (16 bit)/1
  Data Type Conversion111/1 -> M4__mode (8 bit)/1, Display53/1
  Data Type Conversion119/1 -> Display71/1, M4__Motor_hallState (16 bit)/1
  Data Type Conversion118/1 -> Display70/1, M4__Motor_currentPhC (16 bit)/1
  Data Type Conversion110/1 -> Display52/1, M4__status (8 bit)/1
  Data Type Conversion114/1 -> M4__Motor_speed (16 bit)/1, Display50/1
  Data Type Conversion128/1 -> FSR__CH4 (16 bit)/1, Display62/1
  Data Type Conversion129/1 -> FSR__CH5 (16 bit)/1, Display63/1
  Data Type Conversion120/1 -> Display56/1, M4__Motor_dutyCycle (16 bit)/1
  Data Type Conversion126/1 -> FSR__CH2 (16 bit)/1, Display68/1
  Data Type Conversion127/1 -> FSR__CH3 (16 bit)/1, Display69/1
  Data Type Conversion123/1 -> IMU__q_z0 (16 bit)/1, Display61/1
  Data Type Conversion122/1 -> IMU__q_y0 (16 bit)/1, Display60/1
  Data Type Conversion124/1 -> Display58/1, IMU__q_w0 (16 bit)/1
  Data Type Conversion125/1 -> Display59/1, FSR__CH1 (16 bit)/1
  Data Type Conversion121/1 -> IMU__q_x0 (16 bit)/1, Display57/1
  Data Type Conversion130/1 -> Display66/1, Pressure__CH1 (16 bit)/1
  Data Type Conversion131/1 -> Display67/1, Pressure__CH2 (16 bit)/1
  Data Type Conversion132/1 -> Display64/1, Pressure__CH3 (16 bit)/1
  Data Type Conversion71/1 -> Display9/1, M1_Joint_rel_position (16 bit)/1
  Data Type Conversion72/1 -> Display10/1, M1_Joint_abs_position (16 bit)/1
  Data Type Conversion73/1 -> Display11/1, M1__Motor_speed (16 bit)/1
  Data Type Conversion97/1 -> SPARE__3_TX (16 bit)/1, Display31/1
  Data Type Conversion100/1 -> Display32/1, M3__mode (8 bit)/1
  Data Type Conversion113/1 -> Display47/1, M4_Joint_abs_position (16 bit)/1
  Data Type Conversion116/1 -> Display48/1, M4__Motor_currentPhA (16 bit)/1
  Data Type Conversion18/1 -> Display65/1, M1__mode (8 bit)/1
  BLDC Block1/2 -> Data Type Conversion18/1
  Data Type Conversion19/1 -> Display3/1, EMG_CH5 (16 bit)/1
  Data Type Conversion20/1 -> Display4/1, EMG_CH6 (16 bit)/1
  Data Type Conversion21/1 -> Display5/1, EMG_CH7 (16 bit)/1
  Data Type Conversion22/1 -> Display72/1, EMG_CH8 (16 bit)/1
  BLDC Block1/30 -> Data Type Conversion22/1
  BLDC Block1/29 -> Data Type Conversion21/1
  BLDC Block1/28 -> Data Type Conversion20/1
  BLDC Block1/27 -> Data Type Conversion19/1

== matlab function Control_ETHERLAB_2018b/MATLAB Function ==
  data: q input; q_out output; X_d input
function q_out  = Differential_Kinematics(q, X_d)
% Calculates a statistical mean and a standard
% deviation for the values in vals.

l1 = 0.6;
l2 = 0.6;


J = [- l2*sin(q(1) + q(2))-l1*sin(q(1)), -l2*sin(q(1) + q(2)), 0; 
    l2*cos(q(1) + q(2)) + l1*cos(q(1)), l2*cos(q(1) + q(2)), 0
    1,1,1 ];
    if det(J) ~= 0
        delta_q = J\(X_d-ef_pos_from_q(q(1), q(2), q(3), l1, l2));
        q_out = q + delta_q;
    else
        q_out = q;
    end

end


function X = ef_pos_from_q(q1, q2, q3, l1, l2)
%X = [x y phi]
X = [l2*cos(q1 + q2) + l1*cos(q1) l2*sin(q1 + q2) + l1*sin(q1) q1 + q2 + q3]';
end
